simulink model "UnTrans_lin_sim1"  (R2015a)
settings: Solver=ode3  StartTime=0.0  StopTime=10.0  FixedStep=0.01  RelTol=1e-3
values from neighbouring files (symbols this model uses):
  A6 = [0 0 0 0 0 0 1 -0.473294023561 0 0.140107081629 0 0 ... (36 elements, 6x6)]    [ABC_buildin.mat]
  B6 = [0  0; 109.366397902  109.366397902; 0  0; -32.3752383836  -32.3752383836; 0  0; -0.505542240863  0.505542240863]    [ABC_buildin.mat]
  C6 = [1 0 0 0 0 0 0 1 0 0 0 0 ... (36 elements, 6x6)]    [ABC_buildin.mat]
settings Model: CovSFcnEnable=off  Creator=kha  LastModifiedBy=RBoth
settings DataIOCC: SignalLoggingSaveFormat=ModelDataLogs
settings OptimizationCC: ExpressionDepthLimit=2147483647
settings DebuggingCC: UnderspecifiedInitializationDetection=Classic  MergeDetectMultiDrivingBlocksExec=none  SolverPrmCheckMsg=warning  FcnCallInpInsideContextMsg=EnableAllAsWarning  StateNameClashWarn=warning
settings GRTTargetCC: CombineOutputUpdateFcns=off  GRTInterface=on

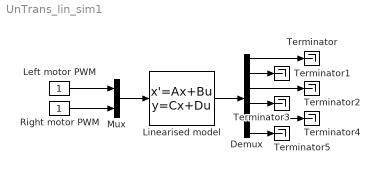
== system UnTrans_lin_sim1 ==
  Demux : Demux  Outputs=6
  Left motor PWM : Constant
  Linearised model : StateSpace  InitFcn=|  A=A6  B=B6  C=C6  D=zeros(6,2)  X0=[0 0 0.1 0 0 0]
      | UnTransPar = UnTransParams( );              
      | [A6, B6, C6] = UnTransLTIModel6(UnTransPar);
      mask Display: image( imread('Trans.jpg','jpg') )
  Mux : Mux  Inputs=2
  Right motor PWM : Constant
  Terminator{,1..5} (6 alike) : Terminator
  wires:
  Mux/1 -> Linearised model/1
  Linearised model/1 -> Demux/1
  Demux/1 -> Terminator/1
  Demux/2 -> Terminator1/1
  Demux/3 -> Terminator2/1
  Demux/4 -> Terminator3/1
  Demux/5 -> Terminator4/1
  Demux/6 -> Terminator5/1
  Left motor PWM/1 -> Mux/1
  Right motor PWM/1 -> Mux/2
